simulink model "L2ADAS"  (R2024b)
settings: Solver=VariableStepAuto  StartTime=0.0  StopTime=10.0  RelTol=1e-3
libraries: simulink x3, ACC_L2 x1, AEB_L2 x1, APA_ x1, ESA_L2 x1
settings DataIOCC: LoadExternalInput=on

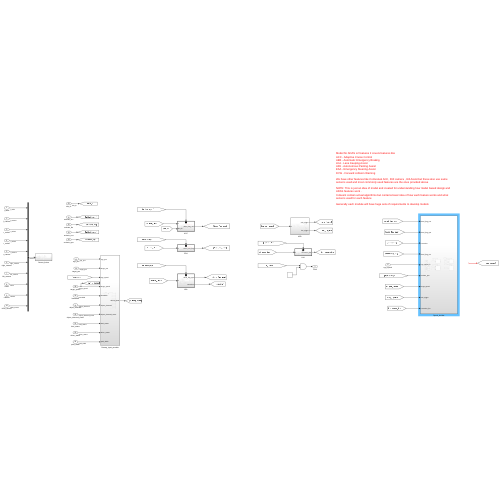
[thumbnail: Simulink's stored preview of the top-level diagram]
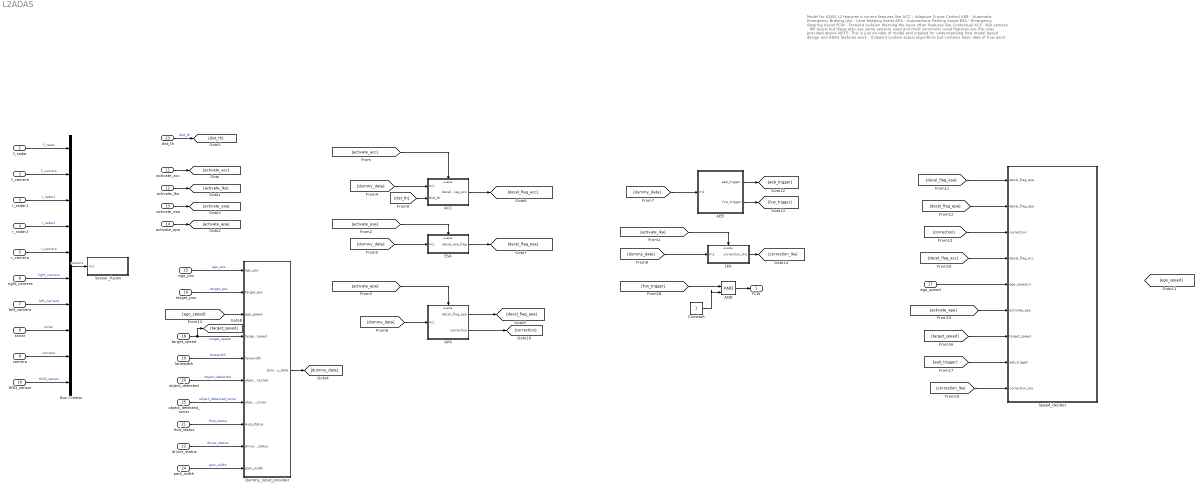
== system L2ADAS ==
  note: Model for ADAS L2 features it covers features like
      | ACC - Adaptive Cruise Control
      | AEB - Automatic Emergency Braking
      | LKA - Lane Keeping Assist
      | APA - Autonomous Parking Assist
      | ESA - Emergency Steering Assist
      | FCW - Forward collision Warning
      |
      | We have other features like Contextual ACC, 360 camera , Hill Assist but these also use same sensors used and most commonly used features are the ones provided above
      |
      | NOTE: This is just an idea of model and created for understanding how model based design and ADAS features work .
      | It doesnt contain actual algorithms but contains basic idea of how each feature works and what sensors used for each feature
      |
      | Generally each module will have huge sets of requirements to develop models
  f_radar : Inport
  f_camera : Inport  Port=2
  r_radar1 : Inport  Port=3
  r_radar2 : Inport  Port=4
  r_camera : Inport  Port=5
  right_camera : Inport  Port=6
  left_camera : Inport  Port=7
  sonar : Inport  Port=8
  camera : Inport  Port=9
  HOD_sensor : Inport  Port=10
  activate_acc : Inport  Port=11  OutDataTypeStr=boolean
  activate_lka : Inport  Port=12  OutDataTypeStr=boolean
  activate_esa : Inport  Port=13  OutDataTypeStr=boolean
  activate_apa : Inport  Port=14  OutDataTypeStr=boolean
  ego_pos : Inport  Port=15
  target_pos : Inport  Port=16
  ego_speed : Inport  Port=17
  target_speed : Inport  Port=18
  lanewidth : Inport  Port=19
  object_detected : Inport  Port=20
  Hod_status : Inport  Port=21
  driver_status : Inport  Port=22
  dist_th : Inport  Port=23
  park_width : Inport  Port=24
  object_detected_sonar : Inport  Port=25
  ACC : Subsystem  TreatAsAtomicUnit=on
  AEB : Subsystem
  AND : Logic  IconShape=distinctive  AllPortsSameDT=off  OutDataTypeStr=boolean
  APA : Subsystem  TreatAsAtomicUnit=on
  Bus Creator : BusCreator  Inputs=10
  Constant : Constant
  Dummy_input_provider : Subsystem
  ESA : Subsystem  TreatAsAtomicUnit=on
  LKA : Subsystem  TreatAsAtomicUnit=on
  Sensor_fusion : Subsystem
  Speed_decider : Subsystem
  FCW : Outport
  wires:
  Bus Creator/1 -> Sensor_fusion/1(In1)  "sensors"
  sonar/1 -> Bus Creator/8  "sonar"
  r_camera/1 -> Bus Creator/5  "r_camera"
  r_radar2/1 -> Bus Creator/4  "r_radar2"
  r_radar1/1 -> Bus Creator/3  "r_radar1"
  f_camera/1 -> Bus Creator/2  "f_camera"
  left_camera/1 -> Bus Creator/7  "left_camera"
  right_camera/1 -> Bus Creator/6  "right_camera"
  f_radar/1 -> Bus Creator/1  "f_radar"
  camera/1 -> Bus Creator/9  "camera"
  HOD_sensor/1 -> Bus Creator/10  "HOD_sensor"
  activate_acc/1 -> [activate_acc]
  activate_lka/1 -> [activate_lka]
  activate_esa/1 -> [activate_esa]
  activate_apa/1 -> [activate_apa]
  [activate_esa] -> ESA/Enable
  [activate_acc] -> ACC/Enable
  [activate_apa] -> APA/Enable
  ego_pos/1 -> Dummy_input_provider/1(ego_pos)  "ego_pos"
  target_pos/1 -> Dummy_input_provider/2(target_pos)  "target_pos"
  target_speed/1 -> Dummy_input_provider/4(target_speed), [target_speed]  "target_speed"
  lanewidth/1 -> Dummy_input_provider/5(lanewidth)  "lanewidth"
  object_detected/1 -> Dummy_input_provider/6(object_detected)  "object_detected"
  Hod_status/1 -> Dummy_input_provider/8(Hod_status)  "Hod_status"
  driver_status/1 -> Dummy_input_provider/9(driver_status)  "driver_status"
  Dummy_input_provider/1(dummy_data) -> [dummy_data]
  [dummy_data] -> ACC/1(In1)
  [dummy_data] -> ESA/1(In1)
  [dummy_data] -> APA/1(In1)
  [dummy_data] -> AEB/1(In1)
  [dummy_data] -> LKA/1(In1)
  dist_th/1 -> [dist_th]  "dist_th"
  [dist_th] -> ACC/2(dist_th)
  ACC/1(decel_flag_acc) -> [decel_flag_acc]
  ESA/1(decel_esa_flag) -> [decel_flag_esa]
  park_width/1 -> Dummy_input_provider/10(park_width)  "park_width"
  APA/1(decel_flag_apa) -> [decel_flag_apa]
  APA/2(correction) -> [correction]
  [decel_flag_esa] -> Speed_decider/1(decel_flag_esa)
  [decel_flag_apa] -> Speed_decider/2(decel_flag_apa)
  [correction] -> Speed_decider/3(correction)
  [decel_flag_acc] -> Speed_decider/4(decel_flag_acc)
  ego_speed/1 -> Speed_decider/5(ego_speed_in)
  ? -> [ego_speed]
  [ego_speed] -> Dummy_input_provider/3(ego_speed)
  [activate_apa] -> Speed_decider/6(activate_apa)
  [target_speed] -> Speed_decider/7(target_speed)
  AEB/1(aeb_trigger) -> [aeb_trigger]
  AEB/2(fcw_trigger) -> [fcw_trigger]
  [aeb_trigger] -> Speed_decider/8(aeb_trigger)
  [fcw_trigger] -> AND/1
  Constant/1 -> AND/2
  AND/1 -> FCW/1
  [activate_lka] -> LKA/Enable
  LKA/1(correction_lka) -> [correction_lka]
  [correction_lka] -> Speed_decider/9(correction_lka)
  object_detected_sonar/1 -> Dummy_input_provider/7(object_detected_sonar)  "object_detected_sonar"

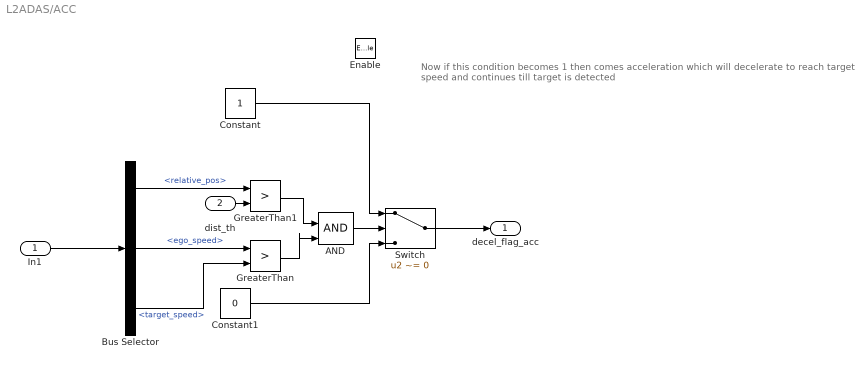
== system L2ADAS/ACC ==
  note: Now if this condition becomes 1 then comes acceleration which will decelerate to reach target speed and continues till target is detected
  In1 : Inport
  dist_th : Inport  Port=2
  Enable : EnablePort  StatesWhenEnabling=reset
  AND : Logic  IconShape=distinctive  AllPortsSameDT=off  OutDataTypeStr=boolean
  Bus Selector : BusSelector  OutputSignals=relative_pos,ego_speed,target_speed
  Constant : Constant
  Constant1 : Constant  Value=0
  GreaterThan : RelationalOperator  Operator=>  OutDataTypeStr=boolean  RndMeth=Simplest  InputSameDT=off
  GreaterThan1 : RelationalOperator  Operator=>  OutDataTypeStr=boolean  RndMeth=Simplest  InputSameDT=off
  Switch : Switch  Criteria=u2 ~= 0  SaturateOnIntegerOverflow=off  InputSameDT=off
  decel_flag_acc : Outport
  wires:
  In1/1 -> Bus Selector/1
  Bus Selector/1 -> GreaterThan1/1  "<relative_pos>"
  dist_th/1 -> GreaterThan1/2
  Bus Selector/2 -> GreaterThan/1  "<ego_speed>"
  Bus Selector/3 -> GreaterThan/2  "<target_speed>"
  AND/1 -> Switch/2
  GreaterThan1/1 -> AND/1
  GreaterThan/1 -> AND/2
  Constant/1 -> Switch/1
  Constant1/1 -> Switch/3
  Switch/1 -> decel_flag_acc/1

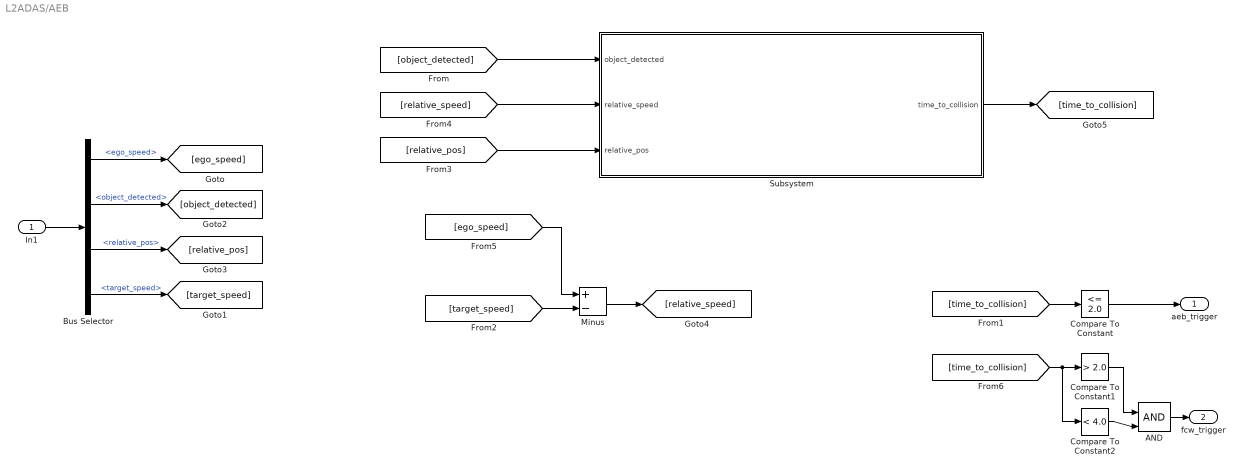
== system L2ADAS/AEB ==
  In1 : Inport
  AND : Logic  IconShape=distinctive  AllPortsSameDT=off  OutDataTypeStr=boolean
  Bus Selector : BusSelector  OutputSignals=ego_speed,object_detected,relative_pos,target_speed
  Compare To Constant : simulink/Logic and Bit Operations/Compare To Constant  relop=<=  const=2.0  OutDataTypeStr=boolean
  Compare To Constant1 : simulink/Logic and Bit Operations/Compare To Constant  relop=>  const=2.0  OutDataTypeStr=boolean
  Compare To Constant2 : simulink/Logic and Bit Operations/Compare To Constant  relop=<  const=4.0  OutDataTypeStr=boolean
  Minus : Sum  Inputs=+-
  Subsystem : Subsystem
  aeb_trigger : Outport
  fcw_trigger : Outport  Port=2
  wires:
  In1/1 -> Bus Selector/1
  Bus Selector/1 -> [ego_speed]  "<ego_speed>"
  Bus Selector/2 -> [object_detected]  "<object_detected>"
  Subsystem/1(time_to_collision) -> [time_to_collision]
  Bus Selector/3 -> [relative_pos]  "<relative_pos>"
  Bus Selector/4 -> [target_speed]  "<target_speed>"
  [ego_speed] -> Minus/1
  [target_speed] -> Minus/2
  Minus/1 -> [relative_speed]
  [relative_speed] -> Subsystem/2(relative_speed)
  [object_detected] -> Subsystem/1(object_detected)
  [relative_pos] -> Subsystem/3(relative_pos)
  [time_to_collision] -> Compare To Constant/1
  Compare To Constant/1 -> aeb_trigger/1
  [time_to_collision] -> Compare To Constant2/1, Compare To Constant1/1
  Compare To Constant2/1 -> AND/2
  Compare To Constant1/1 -> AND/1
  AND/1 -> fcw_trigger/1

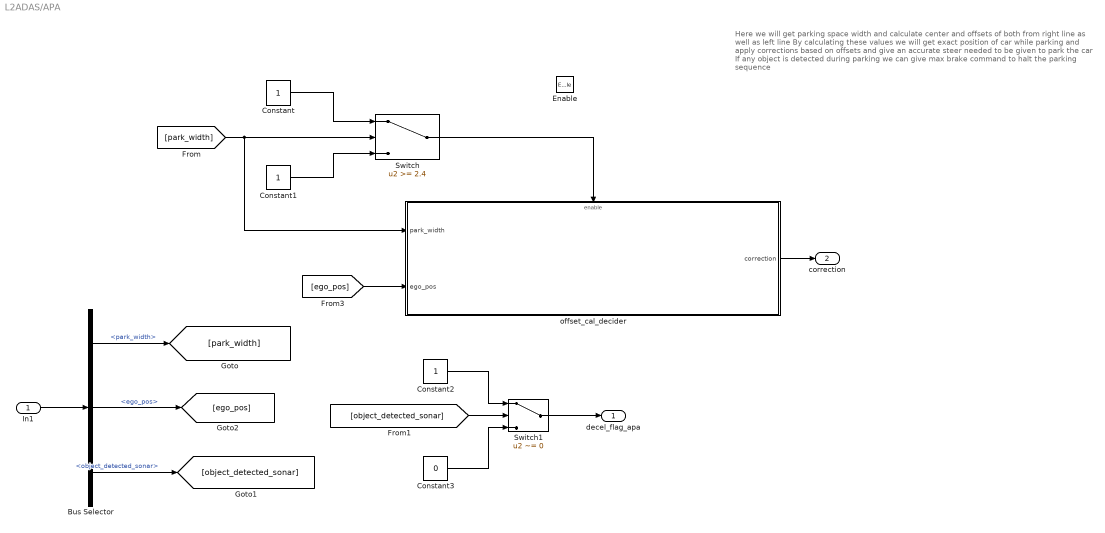
== system L2ADAS/APA ==
  note: Here we will get parking space width and calculate center and offsets of both from right line as well as left line
      | By calculating these values we will get exact position of car while parking and apply corrections based on offsets and give an accurate steer needed to be given to park the car
      | If any object is detected during parking we can give max brake command to halt the parking sequence
  In1 : Inport
  Enable : EnablePort
  Bus Selector : BusSelector  OutputSignals=park_width,ego_pos,object_detected_sonar
  Constant : Constant
  Constant1 : Constant
  Constant2 : Constant
  Constant3 : Constant  Value=0
  Switch : Switch  Threshold=2.4  SaturateOnIntegerOverflow=off  InputSameDT=off
  Switch1 : Switch  Criteria=u2 ~= 0  SaturateOnIntegerOverflow=off  InputSameDT=off
  offset_cal_decider : Subsystem
  decel_flag_apa : Outport
  correction : Outport  Port=2
  wires:
  In1/1 -> Bus Selector/1
  Bus Selector/1 -> [park_width]  "<park_width>"
  Bus Selector/3 -> [object_detected_sonar]  "<object_detected_sonar>"
  Switch/1 -> offset_cal_decider/Enable
  [park_width] -> offset_cal_decider/1(park_width), Switch/2
  Constant/1 -> Switch/1
  Constant1/1 -> Switch/3
  [object_detected_sonar] -> Switch1/2
  Constant2/1 -> Switch1/1
  Constant3/1 -> Switch1/3
  Switch1/1 -> decel_flag_apa/1
  Bus Selector/2 -> [ego_pos]  "<ego_pos>"
  [ego_pos] -> offset_cal_decider/2(ego_pos)
  offset_cal_decider/1(correction) -> correction/1

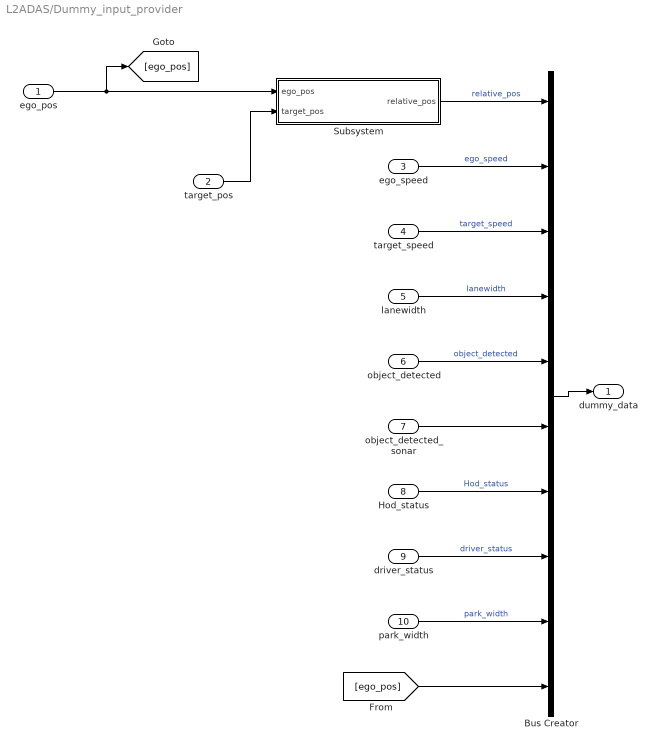
== system L2ADAS/Dummy_input_provider ==
  ego_pos : Inport
  target_pos : Inport  Port=2
  ego_speed : Inport  Port=3
  target_speed : Inport  Port=4
  lanewidth : Inport  Port=5
  object_detected : Inport  Port=6
  object_detected_sonar : Inport  Port=7
  Hod_status : Inport  Port=8
  driver_status : Inport  Port=9
  park_width : Inport  Port=10
  Bus Creator : BusCreator  Inputs=10
  Subsystem : Subsystem
  dummy_data : Outport
  wires:
  Bus Creator/1 -> dummy_data/1
  park_width/1 -> Bus Creator/9  "park_width"
  lanewidth/1 -> Bus Creator/4  "lanewidth"
  target_speed/1 -> Bus Creator/3  "target_speed"
  [ego_pos] -> Bus Creator/10
  ego_speed/1 -> Bus Creator/2  "ego_speed"
  object_detected/1 -> Bus Creator/5  "object_detected"
  Subsystem/1(relative_pos) -> Bus Creator/1  "relative_pos"
  driver_status/1 -> Bus Creator/8  "driver_status"
  Hod_status/1 -> Bus Creator/7  "Hod_status"
  ego_pos/1 -> Subsystem/1(ego_pos), [ego_pos]
  target_pos/1 -> Subsystem/2(target_pos)
  object_detected_sonar/1 -> Bus Creator/6

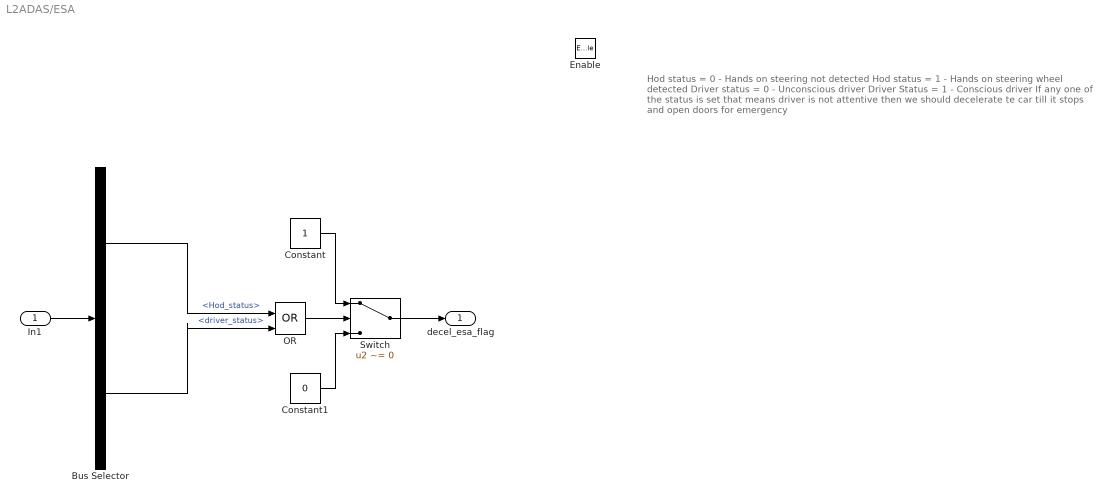
== system L2ADAS/ESA ==
  note: Hod status = 0 - Hands on steering not detected
      |
      | Hod status = 1 - Hands on steering wheel detected
      |
      | Driver status = 0 - Unconscious driver
      |
      | Driver Status = 1 - Conscious driver
      |
      | If any one of the status is set that means driver is not attentive
      | then we should decelerate te car till it stops and open doors for emergency
  In1 : Inport
  Enable : EnablePort
  Bus Selector : BusSelector  OutputSignals=Hod_status,driver_status
  Constant : Constant
  Constant1 : Constant  Value=0
  OR : Logic  Operator=OR  IconShape=distinctive  AllPortsSameDT=off  OutDataTypeStr=boolean
  Switch : Switch  Criteria=u2 ~= 0  SaturateOnIntegerOverflow=off  InputSameDT=off
  decel_esa_flag : Outport
  wires:
  In1/1 -> Bus Selector/1
  OR/1 -> Switch/2
  Bus Selector/1 -> OR/1  "<Hod_status>"
  Bus Selector/2 -> OR/2  "<driver_status>"
  Constant/1 -> Switch/1
  Constant1/1 -> Switch/3
  Switch/1 -> decel_esa_flag/1

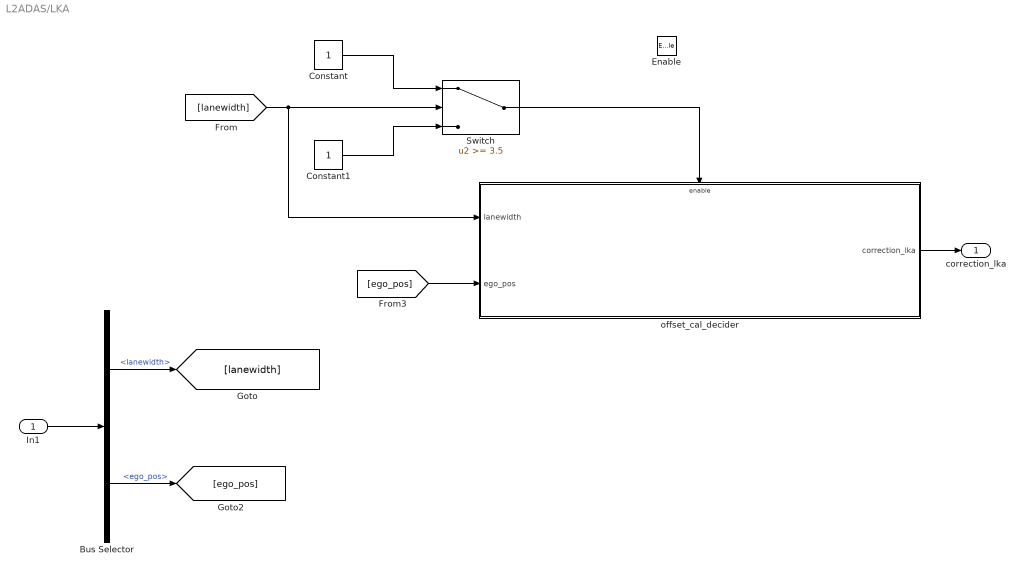
== system L2ADAS/LKA ==
  In1 : Inport
  Enable : EnablePort
  Bus Selector : BusSelector  OutputSignals=lanewidth,ego_pos
  Constant : Constant
  Constant1 : Constant
  Switch : Switch  Threshold=3.5  SaturateOnIntegerOverflow=off  InputSameDT=off
  offset_cal_decider : Subsystem
  correction_lka : Outport
  wires:
  Constant1/1 -> Switch/3
  In1/1 -> Bus Selector/1
  [ego_pos] -> offset_cal_decider/2(ego_pos)
  Switch/1 -> offset_cal_decider/Enable
  offset_cal_decider/1(correction_lka) -> correction_lka/1
  [lanewidth] -> offset_cal_decider/1(lanewidth), Switch/2
  Constant/1 -> Switch/1
  Bus Selector/1 -> [lanewidth]  "<lanewidth>"
  Bus Selector/2 -> [ego_pos]  "<ego_pos>"

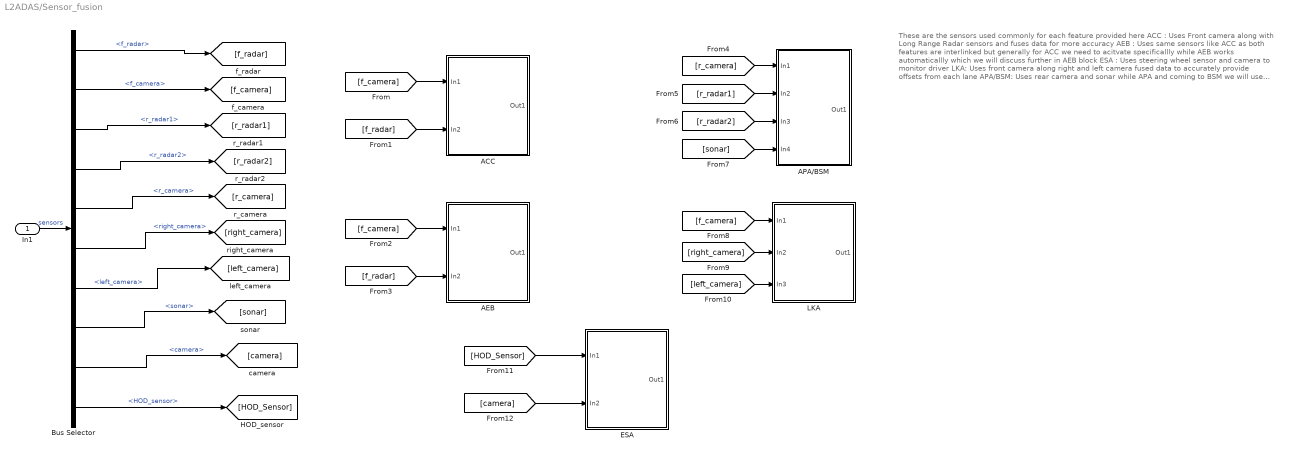
== system L2ADAS/Sensor_fusion ==
  note: These are the sensors used commonly for each feature provided here
      |
      | ACC :
      | Uses Front camera along with Long Range Radar sensors and fuses data for more accuracy
      |
      | AEB :
      | Uses same sensors like ACC as both features are interlinked but generally for ACC we need to acitvate specificallly while AEB works automaticallly which we will discuss further in AEB block
      |
      | ESA :
      | Uses steering wheel sensor and camera to monitor driver
      |
      | LKA:
      | Uses front camera along right and left camera fused data to accurately provide offsets from each lane
      |
      | APA/BSM:
      | Uses rear camera and sonar while APA and coming to BSM we will use medium range radars on both sides of rear for blind spot monitoring along with rear camera
  In1 : Inport
  ACC : Subsystem
  AEB : Subsystem
  APA/BSM : Subsystem
  Bus Selector : BusSelector  OutputSignals=f_radar,f_camera,r_radar1,r_radar2,r_camera,right_camera,left_camera,sonar,camera,HOD_sensor
  ESA : Subsystem
  LKA : Subsystem
  wires:
  Bus Selector/3 -> [r_radar1]  "<r_radar1>"
  Bus Selector/4 -> [r_radar2]  "<r_radar2>"
  Bus Selector/5 -> [r_camera]  "<r_camera>"
  Bus Selector/8 -> [sonar]  "<sonar>"
  Bus Selector/7 -> [left_camera]  "<left_camera>"
  Bus Selector/6 -> [right_camera]  "<right_camera>"
  In1/1 -> Bus Selector/1  "sensors"
  Bus Selector/2 -> [f_camera]  "<f_camera>"
  Bus Selector/1 -> [f_radar]  "<f_radar>"
  [f_camera] -> ACC/1(In1)
  [f_radar] -> ACC/2(In2)
  [f_camera] -> AEB/1(In1)
  [f_radar] -> AEB/2(In2)
  [r_camera] -> APA/BSM/1(In1)
  [r_radar1] -> APA/BSM/2(In2)
  [r_radar2] -> APA/BSM/3(In3)
  [sonar] -> APA/BSM/4(In4)
  [f_camera] -> LKA/1(In1)
  [right_camera] -> LKA/2(In2)
  [left_camera] -> LKA/3(In3)
  Bus Selector/10 -> [HOD_Sensor]  "<HOD_sensor>"
  Bus Selector/9 -> [camera]  "<camera>"
  [HOD_Sensor] -> ESA/1(In1)
  [camera] -> ESA/2(In2)

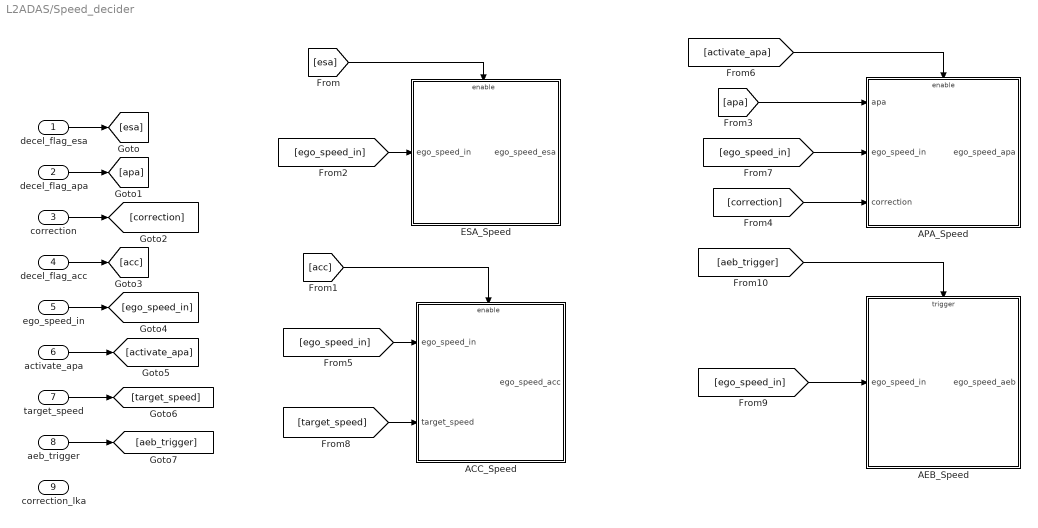
== system L2ADAS/Speed_decider ==
  decel_flag_esa : Inport
  decel_flag_apa : Inport  Port=2
  correction : Inport  Port=3
  decel_flag_acc : Inport  Port=4
  ego_speed_in : Inport  Port=5
  activate_apa : Inport  Port=6
  target_speed : Inport  Port=7
  aeb_trigger : Inport  Port=8
  correction_lka : Inport  Port=9
  ACC_Speed : Subsystem  TreatAsAtomicUnit=on
  AEB_Speed : Subsystem
  APA_Speed : Subsystem  TreatAsAtomicUnit=on
  ESA_Speed : Subsystem  TreatAsAtomicUnit=on
  wires:
  decel_flag_esa/1 -> [esa]
  decel_flag_apa/1 -> [apa]
  correction/1 -> [correction]
  decel_flag_acc/1 -> [acc]
  ego_speed_in/1 -> [ego_speed_in]
  [ego_speed_in] -> ESA_Speed/1(ego_speed_in)
  [esa] -> ESA_Speed/Enable
  [acc] -> ACC_Speed/Enable
  [ego_speed_in] -> ACC_Speed/1(ego_speed_in)
  activate_apa/1 -> [activate_apa]
  [apa] -> APA_Speed/1(apa)
  [activate_apa] -> APA_Speed/Enable
  [ego_speed_in] -> APA_Speed/2(ego_speed_in)
  [correction] -> APA_Speed/3(correction)
  target_speed/1 -> [target_speed]
  [target_speed] -> ACC_Speed/2(target_speed)
  aeb_trigger/1 -> [aeb_trigger]
  [aeb_trigger] -> AEB_Speed/Trigger
  [ego_speed_in] -> AEB_Speed/1(ego_speed_in)

== system L2ADAS/AEB/Subsystem ==
  object_detected : Inport
  relative_speed : Inport  Port=2
  relative_pos : Inport  Port=3
  Enabled Subsystem : Subsystem  TreatAsAtomicUnit=on
  time_to_collision : Outport
  wires:
  object_detected/1 -> Enabled Subsystem/Enable
  relative_pos/1 -> Enabled Subsystem/2(relative_pos)
  relative_speed/1 -> Enabled Subsystem/1(relative_speed)
  Enabled Subsystem/1(time_to_collision) -> time_to_collision/1

== system L2ADAS/APA/offset_cal_decider ==
  park_width : Inport
  ego_pos : Inport  Port=2
  Enable : EnablePort
  offset_calculator : Subsystem
  correction : Outport
  wires:
  park_width/1 -> offset_calculator/1(park_width)
  ego_pos/1 -> offset_calculator/2(ego_pos)
  offset_calculator/1(correction) -> correction/1

== system L2ADAS/Dummy_input_provider/Subsystem ==
  ego_pos : Inport
  target_pos : Inport  Port=2
  Minus : Sum  Inputs=+-
  relative_pos : Outport
  wires:
  ego_pos/1 -> Minus/2
  target_pos/1 -> Minus/1
  Minus/1 -> relative_pos/1

== system L2ADAS/LKA/offset_cal_decider ==
  lanewidth : Inport
  ego_pos : Inport  Port=2
  Enable : EnablePort
  offset_calculator : Subsystem
  correction_lka : Outport
  wires:
  lanewidth/1 -> offset_calculator/1(lanewidth)
  ego_pos/1 -> offset_calculator/2(ego_pos)
  offset_calculator/1(correction_lka) -> correction_lka/1

== system L2ADAS/Sensor_fusion/ACC ==
  In1 : Inport
  In2 : Inport  Port=2
  Out1 : Outport
  wires:
  In1/1 -> Out1/1

== system L2ADAS/Sensor_fusion/AEB ==
  In1 : Inport
  In2 : Inport  Port=2
  Out1 : Outport
  wires:
  In1/1 -> Out1/1

== system L2ADAS/Sensor_fusion/APA//BSM ==
  In1 : Inport
  In2 : Inport  Port=2
  In3 : Inport  Port=3
  In4 : Inport  Port=4
  Out1 : Outport
  wires:
  In1/1 -> Out1/1

== system L2ADAS/Sensor_fusion/ESA ==
  In1 : Inport
  In2 : Inport  Port=2
  Out1 : Outport
  wires:
  In1/1 -> Out1/1

== system L2ADAS/Sensor_fusion/LKA ==
  In1 : Inport
  In2 : Inport  Port=2
  In3 : Inport  Port=3
  Out1 : Outport
  wires:
  In1/1 -> Out1/1

== system L2ADAS/Speed_decider/ACC_Speed ==
  ego_speed_in : Inport
  target_speed : Inport  Port=2
  Enable : EnablePort
  ACC : ACC_L2/ACC  SystemSampleTime=-1  VariantActivationTime=update diagram  AllowFlexibleInterface=on  Latency=0  AutoFrameSizeCalculation=off
  ego_speed_acc : Outport
  wires:
  ACC/1 -> ego_speed_acc/1
  target_speed/1 -> ACC/2
  ego_speed_in/1 -> ACC/1

== system L2ADAS/Speed_decider/AEB_Speed ==
  ego_speed_in : Inport
  Trigger : TriggerPort  VariantControl=(inherit)  PortDimensions=1
  AEB : AEB_L2/AEB  SystemSampleTime=-1  VariantActivationTime=update diagram  AllowFlexibleInterface=on  Latency=0  AutoFrameSizeCalculation=off
  ego_speed_aeb : Outport
  wires:
  AEB/1 -> ego_speed_aeb/1
  ego_speed_in/1 -> AEB/1

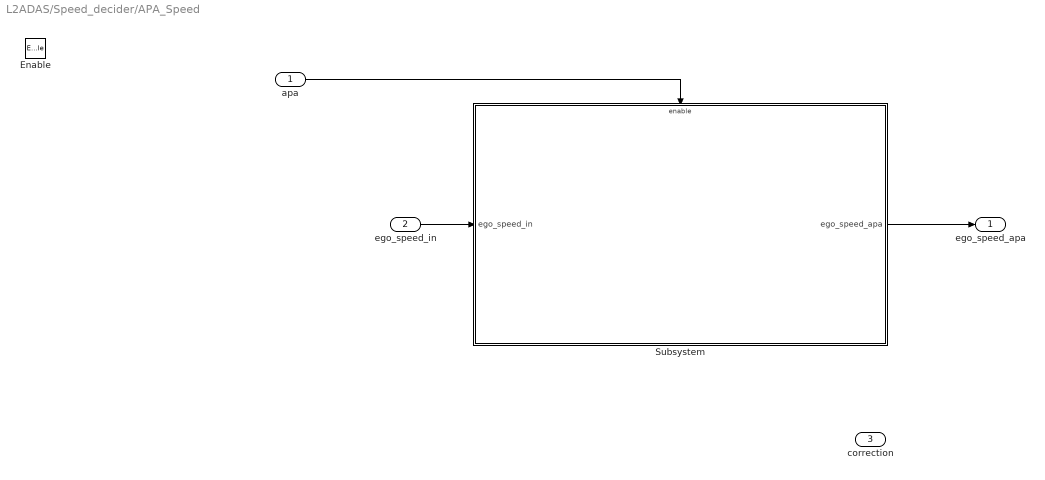
== system L2ADAS/Speed_decider/APA_Speed ==
  apa : Inport
  ego_speed_in : Inport  Port=2
  correction : Inport  Port=3
  Enable : EnablePort
  Subsystem : Subsystem
  ego_speed_apa : Outport
  wires:
  Subsystem/1(ego_speed_apa) -> ego_speed_apa/1
  ego_speed_in/1 -> Subsystem/1(ego_speed_in)
  apa/1 -> Subsystem/Enable

== system L2ADAS/Speed_decider/ESA_Speed ==
  ego_speed_in : Inport
  Enable : EnablePort
  ESA : ESA_L2/ESA  SystemSampleTime=-1  VariantActivationTime=update diagram  AllowFlexibleInterface=on  Latency=0  AutoFrameSizeCalculation=off
  ego_speed_esa : Outport
  wires:
  ego_speed_in/1 -> ESA/1
  ESA/1 -> ego_speed_esa/1

== system L2ADAS/AEB/Subsystem/Enabled Subsystem ==
  relative_speed : Inport
  relative_pos : Inport  Port=2
  object_detected : EnablePort
  Divide : Product  Inputs=*/
  time_to_collision : Outport
  wires:
  relative_pos/1 -> Divide/1
  relative_speed/1 -> Divide/2
  Divide/1 -> time_to_collision/1

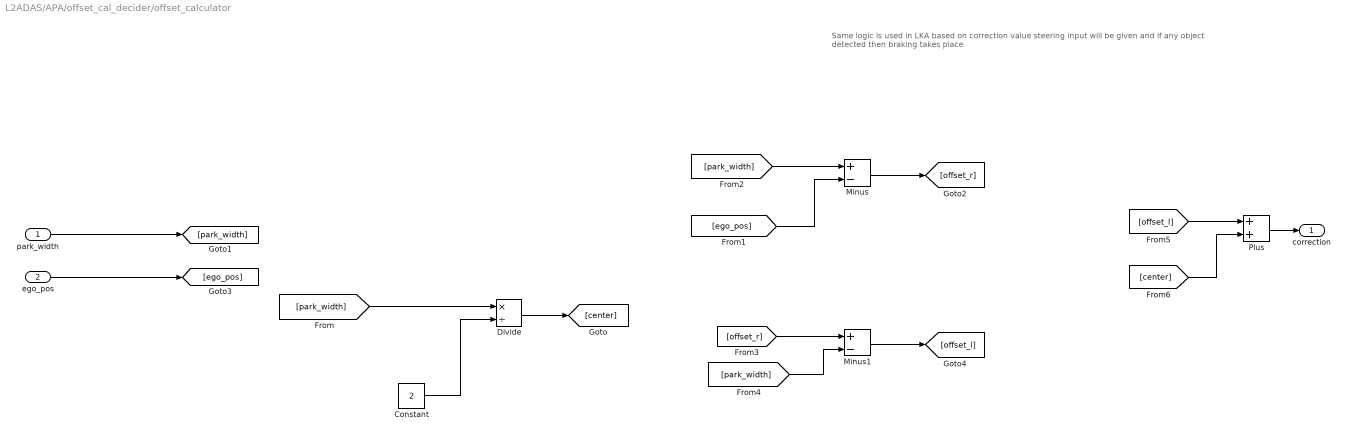
== system L2ADAS/APA/offset_cal_decider/offset_calculator ==
  note: Same logic is used in LKA based on correction value steering input will be given and if any object detected then braking takes place
  park_width : Inport
  ego_pos : Inport  Port=2
  Constant : Constant  Value=2
  Divide : Product  Inputs=*/
  Minus : Sum  Inputs=+-
  Minus1 : Sum  Inputs=+-
  Plus : Sum
  correction : Outport
  wires:
  Constant/1 -> Divide/2
  park_width/1 -> [park_width]
  [park_width] -> Minus/1
  [ego_pos] -> Minus/2
  [park_width] -> Divide/1
  ego_pos/1 -> [ego_pos]
  Divide/1 -> [center]
  Minus/1 -> [offset_r]
  [offset_r] -> Minus1/1
  [park_width] -> Minus1/2
  Minus1/1 -> [offset_l]
  [offset_l] -> Plus/1
  [center] -> Plus/2
  Plus/1 -> correction/1

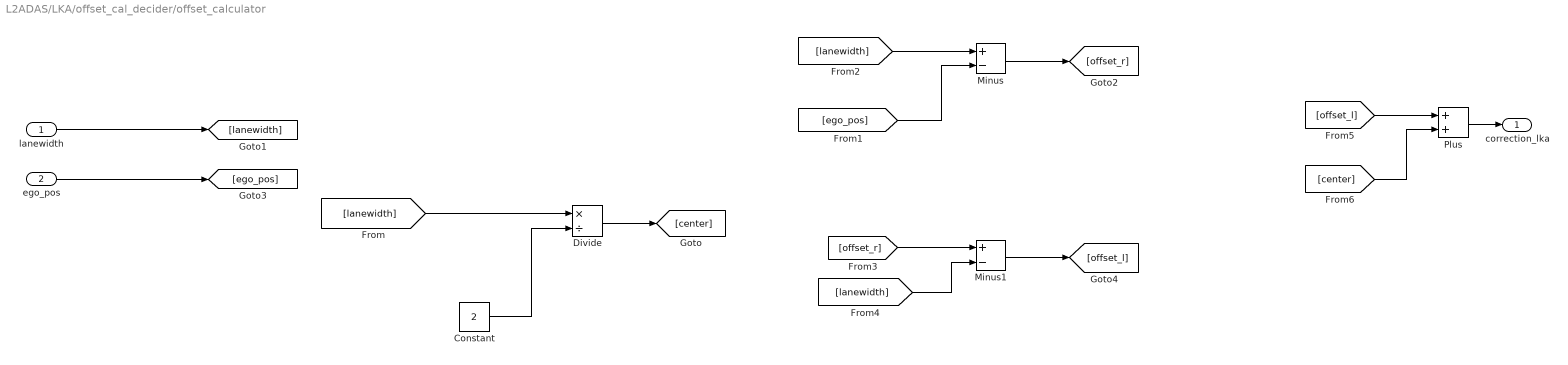
== system L2ADAS/LKA/offset_cal_decider/offset_calculator ==
  lanewidth : Inport
  ego_pos : Inport  Port=2
  Constant : Constant  Value=2
  Divide : Product  Inputs=*/
  Minus : Sum  Inputs=+-
  Minus1 : Sum  Inputs=+-
  Plus : Sum
  correction_lka : Outport
  wires:
  Constant/1 -> Divide/2
  lanewidth/1 -> [lanewidth]
  [lanewidth] -> Minus/1
  [ego_pos] -> Minus/2
  [lanewidth] -> Divide/1
  ego_pos/1 -> [ego_pos]
  Divide/1 -> [center]
  Minus/1 -> [offset_r]
  [offset_r] -> Minus1/1
  [lanewidth] -> Minus1/2
  Minus1/1 -> [offset_l]
  [offset_l] -> Plus/1
  [center] -> Plus/2
  Plus/1 -> correction_lka/1

== system L2ADAS/Speed_decider/APA_Speed/Subsystem ==
  ego_speed_in : Inport
  Enable : EnablePort
  Object_detection_braking : APA_/Object_detection_braking  SystemSampleTime=-1  VariantActivationTime=update diagram  AllowFlexibleInterface=on  Latency=0  AutoFrameSizeCalculation=off
  ego_speed_apa : Outport
  wires:
  ego_speed_in/1 -> Object_detection_braking/1
  Object_detection_braking/1 -> ego_speed_apa/1
